simulink model "clase12012021"  (R2020b)
settings: Solver=VariableStepAuto  StartTime=0.0  StopTime=20/100  RelTol=1e-3
libraries: commdigbbndpm3 x2, dsparch4 x2, commchan3 x1, commsink2 x1, commrandsrc3 x1
settings Model: Creator=fernando  LastModifiedBy=fernando

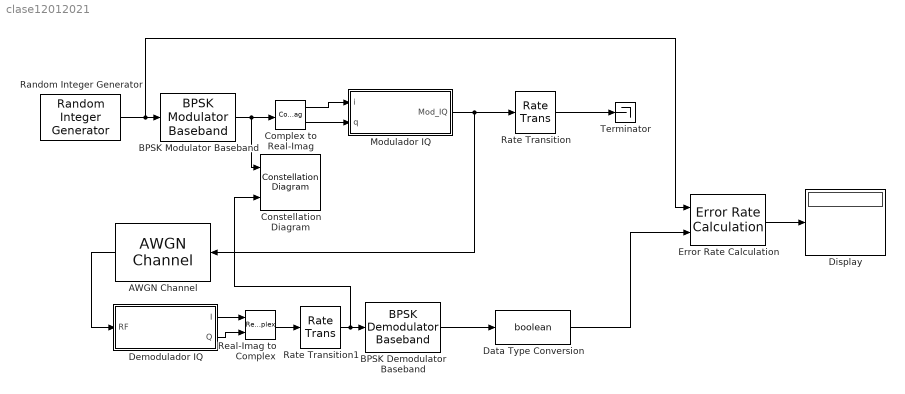
== system clase12012021 ==
  AWGN Channel : commchan3/AWGN Channel  InputProcessing=Columns as channels (frame based)  seed=67  noiseMode="Signal to noise ratio  (Eb/No)"  EbNodB=10  EsNodB=10  SNRdB=10  bitsPerSym=1  Ps=1  Tsym=1  variance=1
  BPSK Demodulator Baseband : commdigbbndpm3/BPSK Demodulator Baseband  DecType=Hard decision  VarSource=Dialog  Variance=1  Ph=0  outDtype=Inherit via internal rule  derotateFactorWordLen=16  derotateFactorDataTypeStr=Inherit: Same word length as input  derotateFactorLastDataTypeStr=Inherit: Same word length as input
      settings: SourceProductName=Communications Toolbox
  BPSK Modulator Baseband : commdigbbndpm3/BPSK Modulator Baseband  Ph=pi/4  outDtype=double  outWordLen=16  outUDDataType=sfix(16)  outFracLenMode=Best precision  outFracLen=15  outDataTypeStr=double  outLastDataTypeStr=double
      settings: SourceProductName=Communications Toolbox
  Complex to Real-Imag : ComplexToRealImag
  Constellation Diagram : ConstellationDiagram  NumInputPorts=2
  Data Type Conversion : DataTypeConversion  OutDataTypeStr=boolean
  Demodulador IQ : Subsystem
  Display : Display
  Error Rate Calculation : commsink2/Error Rate Calculation  N=0  st_delay=0  cp_mode=Entire frame  subframe=[]  PMode=Port  WsName=ErrorVec  RsMode2=off  stop=off  numErr=100  maxBits=1e6
      settings: SourceProductName=Communications Toolbox
  Modulador IQ : Subsystem
  Random Integer Generator : commrandsrc3/Random Integer Generator  SetSize=2  SeedSource=Auto  Seed=0  SampleTime=20/100  SamplesPerFrame=1  OutputDataType=boolean  SimulateUsing=Interpreted execution
  Rate Transition : RateTransition
  Rate Transition1 : RateTransition  OutPortSampleTime=20/100
  Real-Imag to Complex : RealImagToComplex
  Terminator : Terminator
  wires:
  Modulador IQ/1(Mod_IQ) -> AWGN Channel/1, Rate Transition/1
  Complex to Real-Imag/1 -> Modulador IQ/1(i)
  Complex to Real-Imag/2 -> Modulador IQ/2(q)
  BPSK Modulator Baseband/1 -> Constellation Diagram/1, Complex to Real-Imag/1
  Random Integer Generator/1 -> Error Rate Calculation/1, BPSK Modulator Baseband/1
  Rate Transition/1 -> Terminator/1
  Demodulador IQ/1(I) -> Real-Imag to Complex/1
  Demodulador IQ/2(Q) -> Real-Imag to Complex/2
  BPSK Demodulator Baseband/1 -> Data Type Conversion/1
  Rate Transition1/1 -> Constellation Diagram/2, BPSK Demodulator Baseband/1
  Error Rate Calculation/1 -> Display/1
  Data Type Conversion/1 -> Error Rate Calculation/2
  Real-Imag to Complex/1 -> Rate Transition1/1
  AWGN Channel/1 -> Demodulador IQ/1(RF)

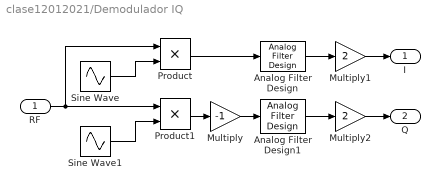
== system clase12012021/Demodulador IQ ==
  RF : Inport
  Analog Filter Design : dsparch4/Analog Filter Design  method=Butterworth  filttype=Lowpass  N=8  Wlo=2*pi*500  Whi=80  Rp=2  Rs=40
  Analog Filter Design1 : dsparch4/Analog Filter Design  method=Butterworth  filttype=Lowpass  N=8  Wlo=2*pi*500  Whi=80  Rp=2  Rs=40
  Multiply : Gain  Gain=-1
  Multiply1 : Gain  Gain=2
  Multiply2 : Gain  Gain=2
  Product : Product
  Product1 : Product
  Sine Wave : Sin  Frequency=2*pi*1e3  SampleTime=0
  Sine Wave1 : Sin  Frequency=2*pi*1e3  SampleTime=0
  I : Outport
  Q : Outport  Port=2
  wires:
  Sine Wave/1 -> Product/2
  RF/1 -> Product1/1, Product/1
  Sine Wave1/1 -> Product1/2
  Product1/1 -> Multiply/1
  Analog Filter Design/1 -> Multiply1/1
  Multiply/1 -> Analog Filter Design1/1
  Product/1 -> Analog Filter Design/1
  Multiply1/1 -> I/1
  Analog Filter Design1/1 -> Multiply2/1
  Multiply2/1 -> Q/1

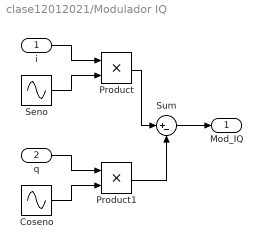
== system clase12012021/Modulador IQ ==
  i : Inport
  q : Inport  Port=2
  Coseno : Sin  Frequency=2*pi*1e3  SampleTime=0
  Product : Product
  Product1 : Product
  Seno : Sin  Frequency=2*pi*1e3  SampleTime=0
  Sum : Sum  Inputs=|+-
  Mod_IQ : Outport
  wires:
  Seno/1 -> Product/2
  i/1 -> Product/1
  Coseno/1 -> Product1/2
  Product1/1 -> Sum/2
  Sum/1 -> Mod_IQ/1
  Product/1 -> Sum/1
  q/1 -> Product1/1
